simulink model "PM_fnc17_ratelimiter5_TestHarness"  (R2022a)
settings: Solver=FixedStepAuto  StartTime=0.0  StopTime=120  FixedStep=rate  RelTol=1e-3
model workspace (MAT data in the model file):
  param_ratelimiter_slewrate_mApermsec = Simulink.Parameter
  param_ratelimiter_slewrate_mApermsec.Value = 10
  param_ratelimiter_slewrate_mApermsec.DataType = 'int32'
  param_ratelimiter_slewrate_mApermsec.Min = 1
  param_ratelimiter_slewrate_mApermsec.Max = 100
  param_ratelimiter_slewrate_mApermsec.DocUnits = 'mA/msec'
  param_ratelimiter_slewrate_mApermsec.Complexity = 'real'
  param_ratelimiter_slewrate_mApermsec.Dimensions = [1 1]
values from neighbouring files (symbols this model uses):
  rate_ms = 10    [PM_fnc1000_tc01_iter01_testsignal_builder.m]    (also in PM_fnc21_tc01_iter01_testsignal_builder.m; PM_fnc22_tc01_iter01_testsignal_builder.m)
undefined symbols (not defined in the file or in its folder): sigbuilder_block, std_lib_block_falling_slew_rate, std_lib_block_rising_slew_rate
settings Model: Creator=306427  LastModifiedBy=306427

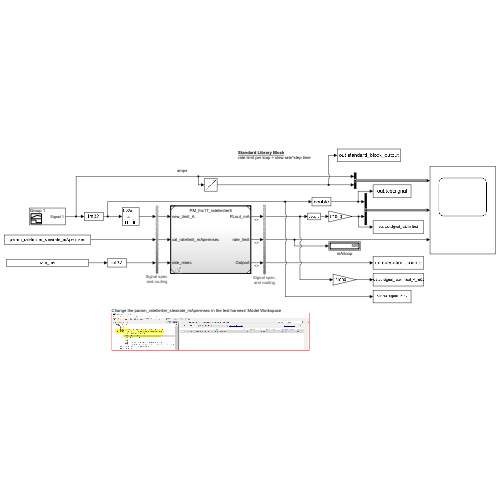
[thumbnail: Simulink's stored preview of the top-level diagram]
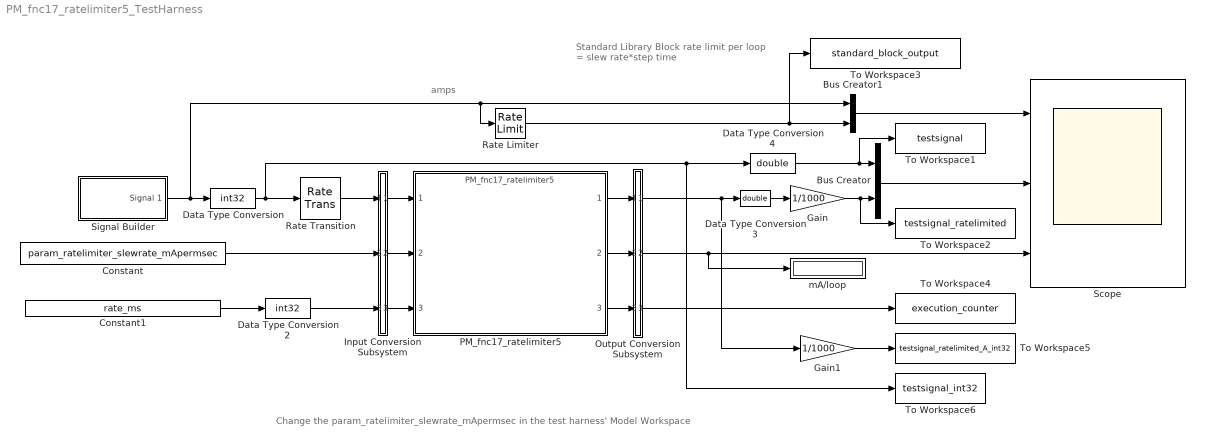
== system PM_fnc17_ratelimiter5_TestHarness ==
  note: Change the param_ratelimiter_slewrate_mApermsec in the test harness' Model Workspace
  note: amps
  note: Standard Library Block
      | rate limit per loop = slew rate*step time
  Bus Creator : BusCreator  Inputs=2
  Bus Creator1 : BusCreator  Inputs=2
  Constant : Constant  Value=param_ratelimiter_slewrate_mApermsec
  Constant1 : Constant  Value=rate_ms
  Data Type Conversion : DataTypeConversion  OutDataTypeStr=int32  SaturateOnIntegerOverflow=off  RndMeth=Floor
  Data Type Conversion2 : DataTypeConversion  OutDataTypeStr=int32  SaturateOnIntegerOverflow=off  RndMeth=Floor
  Data Type Conversion3 : DataTypeConversion  OutDataTypeStr=double  SaturateOnIntegerOverflow=off  RndMeth=Floor
  Data Type Conversion4 : DataTypeConversion  OutDataTypeStr=double  SaturateOnIntegerOverflow=off  RndMeth=Floor
  Gain : Gain  Gain=1/1000
  Gain1 : Gain  Gain=1/1000  OutDataTypeStr=int32
  Input Conversion Subsystem : Subsystem  Tag=__SLT_ICS__  Description=|
      | Signal spec.
      | and routing
      settings: AttributesFormatString=%<Description>
  Output Conversion Subsystem : Subsystem  Tag=__SLT_OCS__  Description=|
      | Signal spec.
      | and routing
      settings: AttributesFormatString=%<Description>
  PM_fnc17_ratelimiter5 : ModelReference  ModelNameDialog=PM_fnc17_ratelimiter5  SimulationMode=Normal  ModelReferenceVersion=1.13
  Rate Limiter : RateLimiter  RisingSlewLimit=std_lib_block_rising_slew_rate  FallingSlewLimit=std_lib_block_falling_slew_rate  SampleTimeMode=inherited
  Rate Transition : RateTransition
  Scope : Scope  NumInputPorts=3
  Signal Builder : Subsystem  Tag=STV Subsys  LoadFcn=sigbuilder_block('load');  StartFcn=sigbuilder_block('start');  StopFcn=sigbuilder_block('stop');  ClipboardFcn=sigbuilder_block('clipboard');  mask(Sigbuilder block){tuvar=[0:10]}
      mask help: Simulink:masks:SigbuilderBlock_MD
      mask init:
      | if ~strcmp(get_param(bdroot(gcbh),'SimulationStatus'),'stopped') tuvar = sigbuilder_block('maskInit'); end
      settings: CopyFcn=sigbuilder_block('copy');  DeleteFcn=sigbuilder_block('delete');  ModelCloseFcn=sigbuilder_block('modelClose');  PreSaveFcn=sigbuilder_block('preSave');  PauseFcn=sigbuilder_block('pause');  ContinueFcn=sigbuilder_block('continue');  NameChangeFcn=sigbuilder_block('namechange');  OpenFcn=sigbuilder_block('open',[537.75 246.75 550.5 359.25 ]);  CloseFcn=sigbuilder_block('close');
      mask Display: plot(0, 0, 100, 100,[2, 2, 32, 32, 2], [68, 8, 8, 68, 68],[32, 2], [38, 38], [32, 19, 2],[53, 60, 44], [32, 17, 17, 2],[16, 16, 31, 31]);txt = getActiveGroup(gcbh);text(2, 100, txt,'verticalAlignment', 'top');
  To Workspace1 : ToWorkspace  VariableName=testsignal  SampleTime=-1
      settings: Save2DSignal=2-D array (concatenate along first dimension)
  To Workspace2 : ToWorkspace  VariableName=testsignal_ratelimited  SampleTime=-1
      settings: Save2DSignal=2-D array (concatenate along first dimension)
  To Workspace3 : ToWorkspace  VariableName=standard_block_output  SampleTime=-1
      settings: Save2DSignal=2-D array (concatenate along first dimension)
  To Workspace4 : ToWorkspace  VariableName=execution_counter  SampleTime=-1
      settings: Save2DSignal=2-D array (concatenate along first dimension)
  To Workspace5 : ToWorkspace  VariableName=testsignal_ratelimited_A_int32  SampleTime=-1
      settings: Save2DSignal=2-D array (concatenate along first dimension)
  To Workspace6 : ToWorkspace  VariableName=testsignal_int32  SampleTime=-1
      settings: Save2DSignal=2-D array (concatenate along first dimension)
  mA/loop : Display
  wires:
  Rate Transition/1 -> Input Conversion Subsystem/1(Inport_1)
  Output Conversion Subsystem/1(Outport_1) -> Gain1/1, Data Type Conversion3/1
  Output Conversion Subsystem/2(Outport_2) -> mA/loop/1, Scope/3
  Gain/1 -> Bus Creator/2, To Workspace2/1
  Data Type Conversion4/1 -> To Workspace1/1, Bus Creator/1
  Data Type Conversion3/1 -> Gain/1
  Rate Limiter/1 -> Bus Creator1/2, To Workspace3/1
  Constant1/1 -> Data Type Conversion2/1
  Bus Creator1/1 -> Scope/1
  Signal Builder/1(Signal 1) -> Bus Creator1/1, Rate Limiter/1, Data Type Conversion/1
  Bus Creator/1 -> Scope/2
  Constant/1 -> Input Conversion Subsystem/2(Inport_2)
  Data Type Conversion2/1 -> Input Conversion Subsystem/3(Inport_3)
  Output Conversion Subsystem/3(Outport_3) -> To Workspace4/1
  Gain1/1 -> To Workspace5/1
  Data Type Conversion/1 -> Rate Transition/1, To Workspace6/1, Data Type Conversion4/1
  PM_fnc17_ratelimiter5/1 -> Output Conversion Subsystem/1(Inport_1)
  PM_fnc17_ratelimiter5/2 -> Output Conversion Subsystem/2(Inport_2)
  PM_fnc17_ratelimiter5/3 -> Output Conversion Subsystem/3(Inport_3)
  Input Conversion Subsystem/1(Outport_1) -> PM_fnc17_ratelimiter5/1
  Input Conversion Subsystem/2(Outport_2) -> PM_fnc17_ratelimiter5/2
  Input Conversion Subsystem/3(Outport_3) -> PM_fnc17_ratelimiter5/3

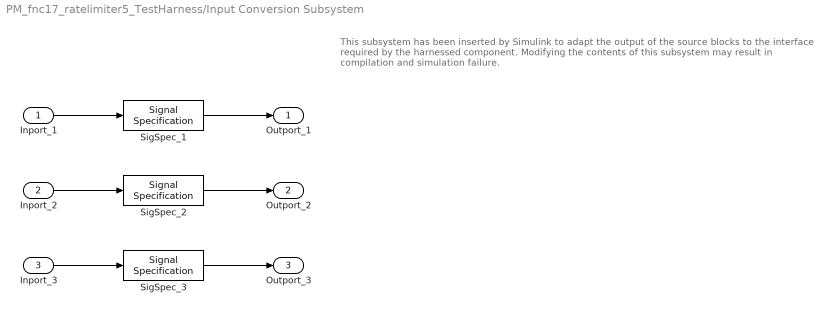
== system PM_fnc17_ratelimiter5_TestHarness/Input Conversion Subsystem ==
  note: This subsystem has been inserted by Simulink to adapt the output of the source blocks to the interface required by the harnessed component.
      |  Modifying the contents of this subsystem may result in compilation and simulation failure.
  Inport_1 : Inport
  Inport_2 : Inport  Port=2
  Inport_3 : Inport  Port=3
  SigSpec_1 : SignalSpecification  OutDataTypeStr=int32  Unit=A  Dimensions=[1, 1]  SampleTime=0.01
  SigSpec_2 : SignalSpecification  OutDataTypeStr=int32  Unit=mA/msec  Dimensions=[1, 1]  SampleTime=0.01
  SigSpec_3 : SignalSpecification  OutDataTypeStr=int32  Unit=msec  Dimensions=[1, 1]  SampleTime=0.01
  Outport_1 : Outport
  Outport_2 : Outport  Port=2
  Outport_3 : Outport  Port=3
  wires:
  SigSpec_1/1 -> Outport_1/1
  Inport_1/1 -> SigSpec_1/1
  SigSpec_2/1 -> Outport_2/1
  Inport_2/1 -> SigSpec_2/1
  SigSpec_3/1 -> Outport_3/1
  Inport_3/1 -> SigSpec_3/1

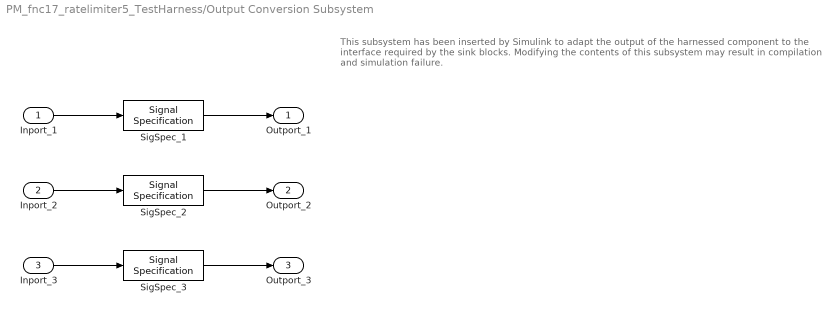
== system PM_fnc17_ratelimiter5_TestHarness/Output Conversion Subsystem ==
  note: This subsystem has been inserted by Simulink to adapt the output of the harnessed component to the interface required by the sink blocks.
      |  Modifying the contents of this subsystem may result in compilation and simulation failure.
  Inport_1 : Inport
  Inport_2 : Inport  Port=2
  Inport_3 : Inport  Port=3
  SigSpec_1 : SignalSpecification  OutDataTypeStr=int32  Unit=mA  Dimensions=[1, 1]  SampleTime=0.01
  SigSpec_2 : SignalSpecification  OutDataTypeStr=int32  Unit=mA/msec  Dimensions=[1, 1]  SampleTime=0.01
  SigSpec_3 : SignalSpecification  OutDataTypeStr=double  Dimensions=[1]  SampleTime=0.01
  Outport_1 : Outport
  Outport_2 : Outport  Port=2
  Outport_3 : Outport  Port=3
  wires:
  Inport_1/1 -> SigSpec_1/1
  SigSpec_1/1 -> Outport_1/1
  Inport_2/1 -> SigSpec_2/1
  SigSpec_2/1 -> Outport_2/1
  Inport_3/1 -> SigSpec_3/1
  SigSpec_3/1 -> Outport_3/1

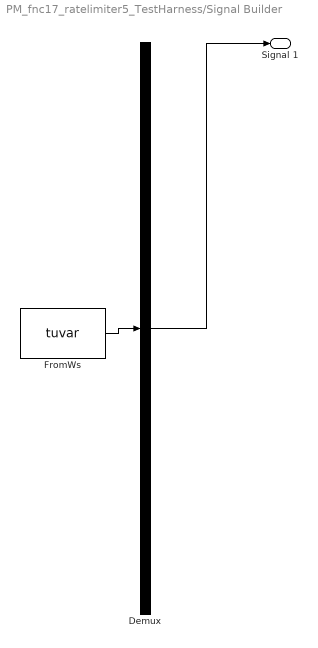
== system PM_fnc17_ratelimiter5_TestHarness/Signal Builder ==
  Demux : Demux  Tag=STV Demux  Outputs=1
      settings: DisplayOption=none
  FromWs : FromWorkspace  Tag=STV FromWs  VariableName=tuvar
      SigBuilderData=|
      | common.afterFinalStr = 'Extrapolate'
      | common.sampleTime = 0
      | dataSet.timeRange = [0 120]
      | dataSet.name = 'Group 1'
      | sbobj.Groups.Name = 'Group 1'
      | sbobj.Groups.Signals.Name = 'Signal 1'
      | sbobj.Groups.Signals.XData = [0 3 3 53 53 120]
      | sbobj.Groups.Signals.YData = [-25 -25 25 25 -25 -25]
      | sbobj.Groups.TimeRange = [0 120]
  Signal 1 : Outport  Tag=STV Outport
  wires:
  FromWs/1 -> Demux/1
  Demux/1 -> Signal 1/1
